simulink model "SOC_Estimation_NN"  (R2022b)
settings: configuration reference "BMS_Sw_CodeGenConfig" (kept outside this file)
undefined symbols (not defined in the file): Np_Module, Ns_Module, NumModules, X_MAX, X_MIN
libraries: deeplib x2
settings Model: DataDictionary=DD_SOC_Estimation.sldd  ExtModeTrigDuration=5  Creator=cpatel  LastModifiedBy=cpatel
settings ConfigSetRef: SourceName=BMS_Sw_CodeGenConfig

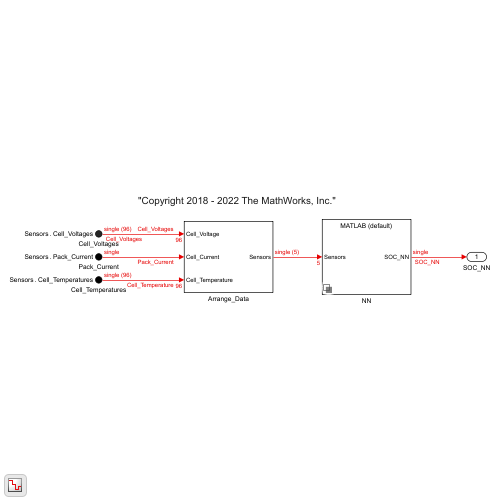
[thumbnail: Simulink's stored preview of the top-level diagram]
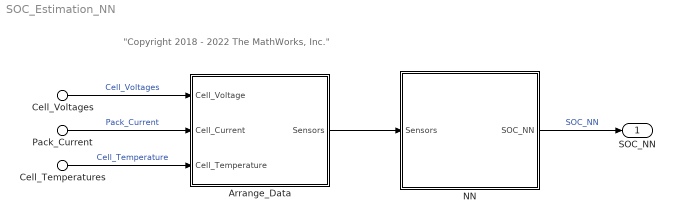
== system SOC_Estimation_NN ==
  note: "Copyright 2018 - 2022 The MathWorks, Inc."
  Cell_Voltages : Inport  PortName=Sensors  Element=Cell_Voltages
  Pack_Current : Inport  PortName=Sensors  Element=Pack_Current
  Cell_Temperatures : Inport  PortName=Sensors  Element=Cell_Temperatures
  Arrange_Data : Subsystem
  NN : Subsystem  Variant=on  VariantControlMode=label  LabelModeActiveChoice=(default)
  SOC_NN : Outport
  wires:
  Cell_Voltages/1 -> Arrange_Data/1(Cell_Voltage)  "Cell_Voltages"
  Pack_Current/1 -> Arrange_Data/2(Cell_Current)  "Pack_Current"
  Cell_Temperatures/1 -> Arrange_Data/3(Cell_Temperature)  "Cell_Temperature"
  NN/1(SOC_NN) -> SOC_NN/1  "SOC_NN"
  Arrange_Data/1(Sensors) -> NN/1(Sensors)

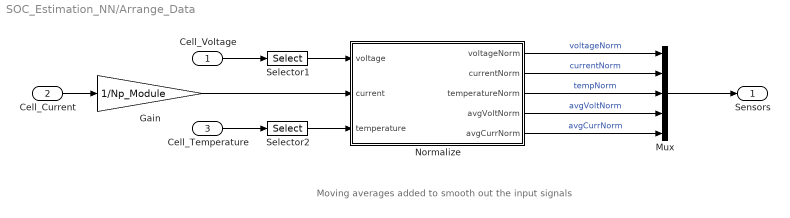
== system SOC_Estimation_NN/Arrange_Data ==
  note: Moving averages added to smooth out the input signals
  Cell_Voltage : Inport
  Cell_Current : Inport  Port=2
  Cell_Temperature : Inport  Port=3
  Gain : Gain  Gain=1/Np_Module
  Mux : Mux  Inputs=5
  Normalize : MATLAB Function  TreatAsAtomicUnit=on
  Selector1 : Selector  InputPortWidth=Ns_Module*NumModules  IndexOptions=Index vector (dialog)  Indices=[1]  OutputSizes=1
  Selector2 : Selector  InputPortWidth=Ns_Module*NumModules  IndexOptions=Index vector (dialog)  Indices=[1]  OutputSizes=1
  Sensors : Outport
  wires:
  Normalize/2(currentNorm) -> Mux/2  "currentNorm"
  Normalize/4(avgVoltNorm) -> Mux/4  "avgVoltNorm"
  Normalize/5(avgCurrNorm) -> Mux/5  "avgCurrNorm"
  Cell_Current/1 -> Gain/1
  Normalize/3(temperatureNorm) -> Mux/3  "tempNorm"
  Cell_Voltage/1 -> Selector1/1
  Mux/1 -> Sensors/1
  Cell_Temperature/1 -> Selector2/1
  Gain/1 -> Normalize/2(current)
  Normalize/1(voltageNorm) -> Mux/1  "voltageNorm"
  Selector2/1 -> Normalize/3(temperature)
  Selector1/1 -> Normalize/1(voltage)

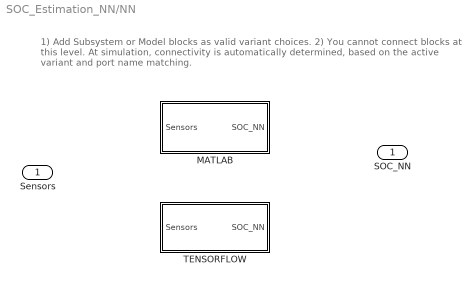
== system SOC_Estimation_NN/NN ==
  note: 1) Add Subsystem or Model blocks as valid variant choices.
      | 2) You cannot connect blocks at this level. At simulation, connectivity is automatically
      | determined, based on the active variant and port name matching.
  Sensors : Inport
  MATLAB : Subsystem  VariantControl=(default)
  TENSORFLOW : Subsystem  VariantControl=TF
  SOC_NN : Outport

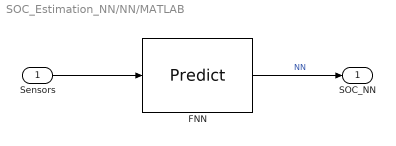
== system SOC_Estimation_NN/NN/MATLAB ==
  Sensors : Inport
  FNN : deeplib/Predict  Network=Network from MAT-file  NetworkFunction=squeezenet  NetworkFilePath=net.mat  MiniBatchSize=1  InputDataFormats={ '', '' }  Predictions=on  Activations={}  ForceInterpretedSim=off  EnableDLNetwork=off
  SOC_NN : Outport
  wires:
  FNN/1 -> SOC_NN/1  "NN"
  Sensors/1 -> FNN/1

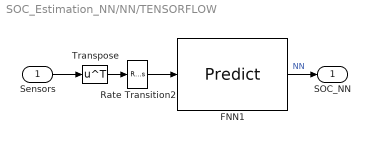
== system SOC_Estimation_NN/NN/TENSORFLOW ==
  Sensors : Inport
  FNN1 : deeplib/Predict  Network=Network from MAT-file  NetworkFunction=squeezenet  NetworkFilePath=battery_S0C_net_TF.mat  MiniBatchSize=1  InputDataFormats={ '', '' }  Predictions=on  Activations={}  ForceInterpretedSim=off  EnableDLNetwork=off
  Rate Transition2 : RateTransition  OutPortSampleTime=1
  Transpose : Math  Operator=transpose
  SOC_NN : Outport
  wires:
  Rate Transition2/1 -> FNN1/1
  Transpose/1 -> Rate Transition2/1
  FNN1/1 -> SOC_NN/1  "NN"
  Sensors/1 -> Transpose/1

== matlab function SOC_Estimation_NN/Arrange_Data/Normalize ==
  data: voltage input; current input; temperature input; voltageNorm output; X_MAX parameter; X_MIN parameter; currentNorm output; temperatureNorm output; avgVoltNorm output; avgCurrNorm output
function [voltageNorm ,currentNorm ,temperatureNorm, avgVoltNorm, avgCurrNorm]    = fcn(voltage, current, temperature,X_MAX, X_MIN)

persistent voltNormArray currNormArray

if isempty(voltNormArray)
    voltNormArray = single(zeros(1,400));
end

if isempty(currNormArray)
    currNormArray = single(zeros(1,400));
end

voltageNorm = (voltage - X_MIN(1))./(X_MAX(1) - X_MIN(1));
currentNorm = (current - X_MIN(2))./(X_MAX(2) - X_MIN(2));
temperatureNorm = (temperature - X_MIN(3))./(X_MAX(3) - X_MIN(3));

voltNormArray = circshift(voltNormArray,1);
voltNormArray(1) = voltageNorm;

currNormArray = circshift(currNormArray,1);
currNormArray(1) = currentNorm;

avgVoltNorm = mean(voltNormArray);
avgCurrNorm = mean(currNormArray);


%y = (u - X_MIN)./(X_MAX - X_MIN);
